simulink model "slider_mode_controller_sim_21"  (R2021b)
settings: Solver=VariableStepAuto  StartTime=0.0  StopTime=120  RelTol=1e-3
undefined symbols (not defined in the file): sim_r
settings Model: Creator=alefr  LastModifiedBy=alefr
settings DataIOCC: ReturnWorkspaceOutputs=off

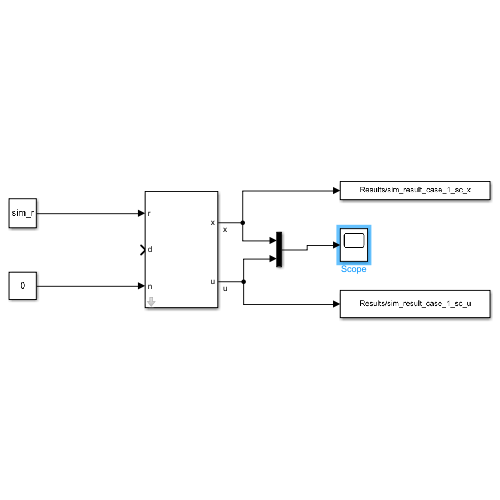
[thumbnail: Simulink's stored preview of the top-level diagram]
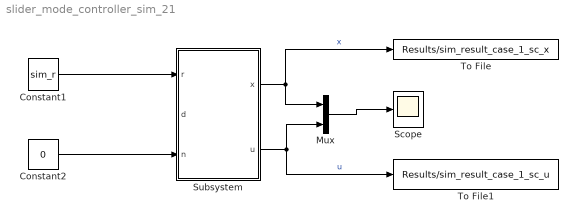
== system slider_mode_controller_sim_21 ==
  Constant1 : Constant  Value=sim_r
  Constant2 : Constant  Value=0
  Mux : Mux  Inputs=2
  Scope : Scope
  Subsystem : Subsystem  mask{p1_param=0.1, p2_param=0.1, epsi_param=0.2, mu_param=0.12, init_state_param=[8;8]}
      mask prompts: p1_param "p1"; p2_param "p2"; epsi_param "epsi"; mu_param "mu"
  To File : ToFile  Filename=Results/sim_result_case_1_sc_x  MatrixName=sim_result_case_1_sc_x  SaveFormat=Timeseries
  To File1 : ToFile  Filename=Results/sim_result_case_1_sc_u  MatrixName=sim_result_case_1_sc_u  SaveFormat=Timeseries
  wires:
  Constant1/1 -> Subsystem/1(r)
  Constant2/1 -> Subsystem/3(n)
  Subsystem/1(x) -> To File/1, Mux/1  "x"
  Subsystem/2(u) -> Mux/2, To File1/1  "u"
  Mux/1 -> Scope/1

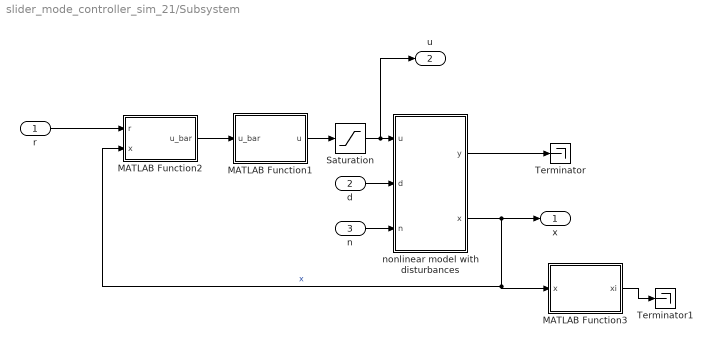
== system slider_mode_controller_sim_21/Subsystem ==
  r : Inport
  d : Inport  Port=2
  n : Inport  Port=3
  MATLAB Function1 : MATLAB Function  TreatAsAtomicUnit=on
  MATLAB Function2 : MATLAB Function  TreatAsAtomicUnit=on
  MATLAB Function3 : MATLAB Function  TreatAsAtomicUnit=on
  Saturation : Saturate  UpperLimit=10  LowerLimit=0
  Terminator : Terminator
  Terminator1 : Terminator
  nonlinear model with disturbances : Subsystem
  x : Outport
  u : Outport  Port=2
  wires:
  nonlinear model with disturbances/2(x) -> MATLAB Function3/1(x), MATLAB Function2/2(x), x/1  "x"
  MATLAB Function3/1(xi) -> Terminator1/1
  nonlinear model with disturbances/1(y) -> Terminator/1
  d/1 -> nonlinear model with disturbances/2(d)
  MATLAB Function2/1(u_bar) -> MATLAB Function1/1(u_bar)
  n/1 -> nonlinear model with disturbances/3(n)
  MATLAB Function1/1(u) -> Saturation/1
  Saturation/1 -> u/1, nonlinear model with disturbances/1(u)
  r/1 -> MATLAB Function2/1(r)

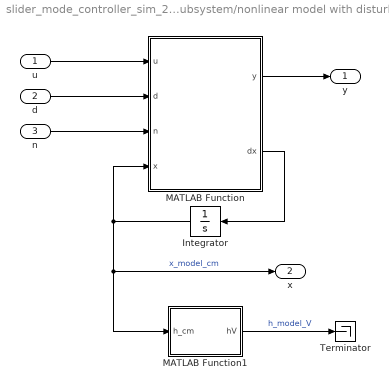
== system slider_mode_controller_sim_21/Subsystem/nonlinear model with disturbances ==
  u : Inport
  d : Inport  Port=2
  n : Inport  Port=3
  Integrator : Integrator  InitialCondition=init_state_param
  MATLAB Function : MATLAB Function  TreatAsAtomicUnit=on
  MATLAB Function1 : MATLAB Function  TreatAsAtomicUnit=on
  Terminator : Terminator
  y : Outport
  x : Outport  Port=2
  wires:
  MATLAB Function/1(y) -> y/1
  n/1 -> MATLAB Function/3(n)
  MATLAB Function1/1(hV) -> Terminator/1  "h_model_V"
  d/1 -> MATLAB Function/2(d)
  MATLAB Function/2(dx) -> Integrator/1
  Integrator/1 -> MATLAB Function/4(x), MATLAB Function1/1(h_cm), x/1  "x_model_cm"
  u/1 -> MATLAB Function/1(u)

== matlab function slider_mode_controller_sim_21/Subsystem/MATLAB Function2 ==
  data: r input; u_bar output; x input; mu_param parameter; p1_param parameter; p2_param parameter; epsi_param parameter
function u_bar = fcn(r,x, mu_param, p1_param, p2_param, epsi_param)

mu = mu_param;
epsi = epsi_param;
p1 = p1_param;
p2 = p2_param;

x1=x(1);
x2=x(2);

u_bar = ((p2.*(sqrt(x1.*5.0+1.6e+1).*7.609042393596842e-2-sqrt(x2.*5.0+1.6e+1).*7.609042393596842e-2).*1.0./sqrt(abs(p1).^2+abs(p2).^2)+p1.*1.0./sqrt(x1.*5.0+1.6e+1).*1.0./sqrt(x2.*5.0+1.6e+1).*(x1.*2.7795e+4+8.8944e+4).*1.0./sqrt(abs(p1).^2+abs(p2).^2).*3.491988616282361e-6).*sqrt(x1.*5.0+1.6e+1).*sqrt(abs(p1).^2+abs(p2).^2).*(-1.734778086018821e+2))./p1-(mu.*sqrt(x1.*5.0+1.6e+1).*sqrt(abs(p1).^2+abs(p2).^2).*min([1.0,max([-1.0,(p1.*(sqrt(x1.*1.962e+3+6.2784e+3).*3.841187477910597e-3-sqrt(x2.*1.962e+3+6.2784e+3).*3.841187477910597e-3)-p2.*(r-x2.*7.456422751238219e-1+1.648066384406454))./epsi],[],2,'omitnan')],[],2,'omitnan').*1.734778086018821e+2)./p1;


end

== matlab function slider_mode_controller_sim_21/Subsystem/MATLAB Function1 ==
  data: u_bar input; u output
function u = pm1(u_bar)

u = u_bar.*3.277899884284337e-1-u_bar.^2.*9.88758313621772e-3+u_bar.^3.*1.567756031883916e-4-2.914041336753123;

end

== matlab function slider_mode_controller_sim_21/Subsystem/MATLAB Function3 ==
  data: x input; xi output
function xi = T(x)

x1 = x(1);
x2 = x(2);

xi = [x2.*7.456422751238219e-1-1.648066384406454;sqrt(x1.*1.962e+3+6.2784e+3).*3.841187477910597e-3-sqrt(x2.*1.962e+3+6.2784e+3).*3.841187477910597e-3];

end

== matlab function slider_mode_controller_sim_21/Subsystem/nonlinear model with disturbances/MATLAB Function ==
  data: y output; u input; dx output; d input; n input; x input
function [y,dx] = nonlinear_model(u,d,n,x)

x1 = x(1);
x2 = x(2);

y = x2.*7.456422751238219e-1 + n -1.648066384406454;

dx = [+u.*2.81859116712929e-1-(d.*sqrt(x1.*1.962e+3+6.2784e+3))./3.3e+1-sqrt(x1.*1.962e+3+6.2784e+3).*5.151515151515152e-3-u.^2.*2.476601319356692e-2+u.^3.*8.808489605974731e-4+3.751072019731428e-1;sqrt(x1.*1.962e+3+6.2784e+3).*5.151515151515152e-3-sqrt(x2.*1.962e+3+6.2784e+3).*5.151515151515152e-3];

end

== matlab function slider_mode_controller_sim_21/Subsystem/nonlinear model with disturbances/MATLAB Function1 ==
  data: h_cm input; hV output
function hV = g(h_cm)

hV = h_cm*7.456422751238219e-1 - 1.648066384406454;
